simulink model "dextair_mechanics_without_spring"  (R2018b)
settings: Solver=VariableStepAuto  StartTime=0.0  StopTime=100  RelTol=1e-3  EnableMultiTasking=on
values from neighbouring files (symbols this model uses):
  a = 1.7*10^(-6)    (= 1.7e-06)    [MAIN.m]
  delta = 0.32    [MAIN.m]
  g = 9.8    [MAIN.m]
  k = 0    [MAIN.m]
  L = 0.16    [MAIN.m]
  l_0 = 10    [MAIN.m]
  m = 2.07    [MAIN.m]
  PID_D_phi = PID_D    (= 19)    [MAIN.m]
  PID_D_psi = PID_D    (= 19)    [MAIN.m]
  PID_D_theta = PID_D    (= 19)    [MAIN.m]
  PID_D_x = PID_D    (= 19)    [MAIN.m]
  PID_D_y = PID_D    (= 19)    [MAIN.m]
  PID_D_z = PID_D    (= 19)    [MAIN.m]
  PID_I_phi = PID_I    (= 2.12)    [MAIN.m]
  PID_I_psi = PID_I    (= 2.12)    [MAIN.m]
  PID_I_theta = PID_I    (= 2.12)    [MAIN.m]
  PID_I_x = PID_I    (= 2.12)    [MAIN.m]
  PID_I_y = PID_I    (= 2.12)    [MAIN.m]
  PID_I_z = PID_I    (= 2.12)    [MAIN.m]
  PID_P_phi = PID_P    (= 12.71)    [MAIN.m]
  PID_P_psi = PID_P    (= 12.71)    [MAIN.m]
  PID_P_theta = PID_P    (= 12.71)    [MAIN.m]
  PID_P_x = PID_P    (= 12.71)    [MAIN.m]
  PID_P_y = PID_P    (= 12.71)    [MAIN.m]
  PID_P_z = PID_P    (= 12.71)    [MAIN.m]
  s = tf('s')    [MAIN.m]
  xl = 0.01    [MAIN.m]
  Z_0 = m*g/k+l_0    [MAIN.m]
undefined symbols (not defined in the file or in its folder): X, Y, Z
libraries: sm_lib x28, nesl_utility x11, simulink x7
(part 1 of 2)
settings Model: Creator=shaabang  LastModifiedBy=shaabang
settings DataIOCC: LimitDataPoints=on
settings OptimizationCC: LifeSpan=inf
settings DebuggingCC: AllowSymbolicDim=off  SFUnexpectedBacktrackingDiag=warning  SFNoUnconditionalDefaultTransitionDiag=warning  SFExecutionAtInitializationDiag=none
settings SFSimCC: SimUseLocalCustomCode=off
settings RTWCC: RTWUseLocalCustomCode=off
settings CodeAppCC: StateflowObjectComments=on
settings GRTTargetCC: TargetLangStandard=C89/C90 (ANSI)  GeneratePreprocessorConditionals=Disable all
settings ConfigComp: CovMetricSettings=dw  CovHtmlReporting=on  CovSaveCumulativeToWorkspaceVar=on  CovSaveSingleToWorkspaceVar=on  CovExternalEMLEnable=off  CovSFcnEnable=off
settings SimscapeCC: SimscapeNominalValues="[{\"value\":\"10\",\"unit\":\"V\"},{\"value\":\"1\",\"unit\":\"A\"},{\"value\":\"10\",\"unit\":\"N*m\"},{\"value\":\"10\",\"unit\":\"bar\"},{\"value\":\"100\",\"unit\":\"kJ/kg\"},{\"value\":\"1\",\"unit\":\"kW\"},{\"value\":\"300\",\"unit\":\"K\"},{\"value\":\"100\",\"unit\":\"cm^3/s\"},{\"value\":\"1\",\"unit\":\"kN\"},{\"value\":\"1\",\"unit\":\"g/cm^3\"},{\"value\":\"1\",\"unit\":\"l\"},{\"value\":\"1\",\"unit\":\"cm^2\"},{\"value\":\"60\",\"unit\":\"Hz\"}]"  SimscapeLogType=all  SimscapeLogDataHistory=10000
settings ConfigurationSet: Description=SimMechanics 2G

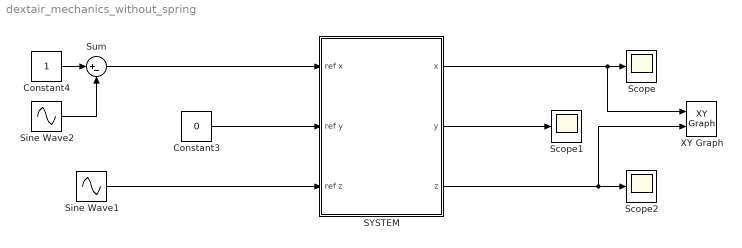
== system dextair_mechanics_without_spring ==
  Constant3 : Constant  Value=0
  Constant4 : Constant
  SYSTEM : Subsystem
  Scope : Scope
  Scope1 : Scope
  Scope2 : Scope
  Sine Wave1 : Sin  Frequency=0.5  SampleTime=0
  Sine Wave2 : Sin  Frequency=0.5  Phase=pi/2  SampleTime=0
  Sum : Sum  Inputs=|+-
  XY Graph : simulink/Sinks/XY Graph  xmin=-0.5  xmax=2.5  ymin=-1.5  ymax=1.5  st=-1
  wires:
  Sum/1 -> SYSTEM/1(ref x)
  SYSTEM/1(x) -> XY Graph/1, Scope/1
  Sine Wave1/1 -> SYSTEM/3(ref z)
  SYSTEM/2(y) -> Scope1/1
  Constant4/1 -> Sum/1
  Constant3/1 -> SYSTEM/2(ref y)
  SYSTEM/3(z) -> XY Graph/2, Scope2/1
  Sine Wave2/1 -> Sum/2

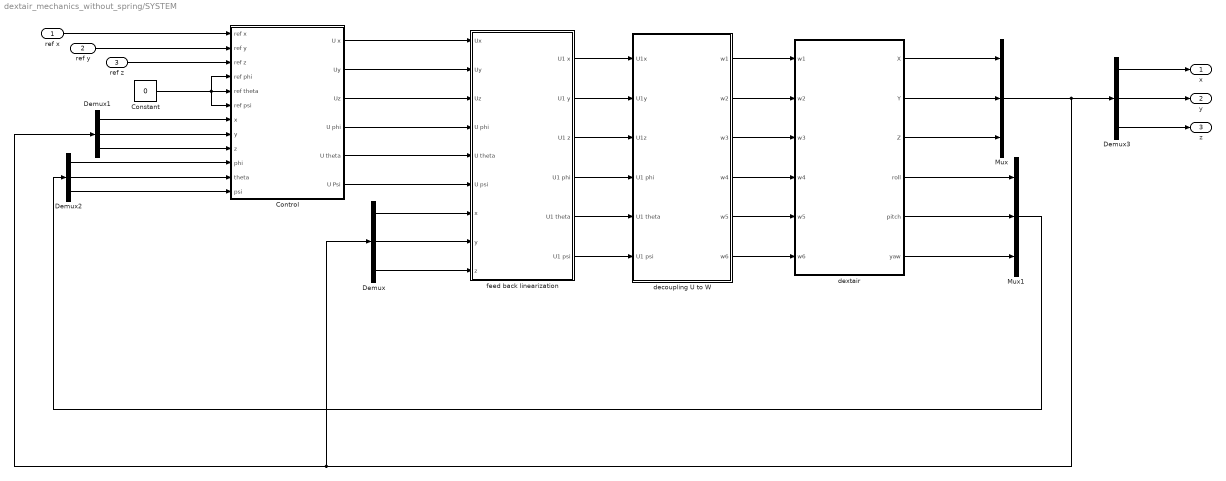
== system dextair_mechanics_without_spring/SYSTEM ==
  ref x : Inport
  ref y : Inport  Port=2
  ref z : Inport  Port=3
  Constant : Constant  Value=0
  Control : Subsystem
  Demux{,1..3} (4 alike) : Demux  Outputs=3
  Mux : Mux  Inputs=3
  Mux1 : Mux  Inputs=3
  decoupling U to W : Subsystem
  dextair : Subsystem
  feed back linearization : Subsystem
  x : Outport
  y : Outport  Port=2
  z : Outport  Port=3
  wires:
  decoupling U to W/5(w5) -> dextair/5(w5)
  Demux1/2 -> Control/8(y)
  feed back linearization/2(U1 y) -> decoupling U to W/2(U1y)
  ref y/1 -> Control/2(ref y)
  Control/2(Uy) -> feed back linearization/2(Uy)
  feed back linearization/5(U1 theta) -> decoupling U to W/5(U1 theta)
  decoupling U to W/2(w2) -> dextair/2(w2)
  decoupling U to W/4(w4) -> dextair/4(w4)
  dextair/5(pitch) -> Mux1/2
  Control/6(U Psi) -> feed back linearization/6(U psi)
  dextair/1(X) -> Mux/1
  Control/5(U theta) -> feed back linearization/5(U theta)
  Demux2/2 -> Control/11(theta)
  decoupling U to W/6(w6) -> dextair/6(w6)
  feed back linearization/3(U1 z) -> decoupling U to W/3(U1z)
  Demux1/1 -> Control/7(x)
  Demux2/3 -> Control/12(psi)
  decoupling U to W/1(w1) -> dextair/1(w1)
  Demux/1 -> feed back linearization/7(x)
  Control/4(U phi) -> feed back linearization/4(U phi)
  Control/3(Uz) -> feed back linearization/3(Uz)
  Constant/1 -> Control/6(ref psi), Control/4(ref phi), Control/5(ref theta)
  Demux2/1 -> Control/10(phi)
  dextair/4(roll) -> Mux1/1
  Demux1/3 -> Control/9(z)
  dextair/6(yaw) -> Mux1/3
  Control/1(U x) -> feed back linearization/1(Ux)
  feed back linearization/6(U1 psi) -> decoupling U to W/6(U1 psi)
  ref x/1 -> Control/1(ref x)
  dextair/3(Z) -> Mux/3
  ref z/1 -> Control/3(ref z)
  Demux3/2 -> y/1
  Demux/2 -> feed back linearization/8(y)
  Demux3/3 -> z/1
  Demux3/1 -> x/1
  dextair/2(Y) -> Mux/2
  feed back linearization/1(U1 x) -> decoupling U to W/1(U1x)
  feed back linearization/4(U1 phi) -> decoupling U to W/4(U1 phi)
  Demux/3 -> feed back linearization/9(z)
  decoupling U to W/3(w3) -> dextair/3(w3)
  Mux1/1 -> Demux2/1
  Mux/1 -> Demux/1, Demux1/1, Demux3/1

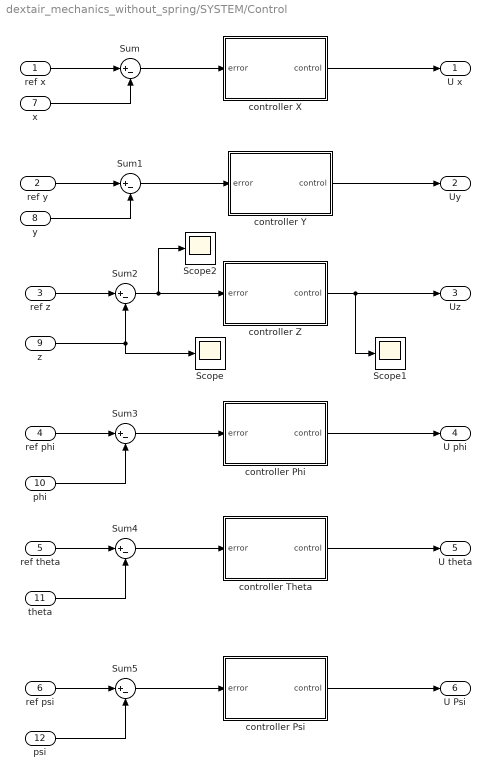
== system dextair_mechanics_without_spring/SYSTEM/Control ==
  ref x : Inport
  ref y : Inport  Port=2
  ref z : Inport  Port=3
  ref phi : Inport  Port=4
  ref theta : Inport  Port=5
  ref psi : Inport  Port=6
  x : Inport  Port=7
  y : Inport  Port=8
  z : Inport  Port=9
  phi : Inport  Port=10
  theta : Inport  Port=11
  psi : Inport  Port=12
  Scope : Scope
  Scope1 : Scope
  Scope2 : Scope
  Sum{,1..5} (6 alike) : Sum  Inputs=|+-
  controller Phi : Subsystem
  controller Psi : Subsystem
  controller Theta : Subsystem
  controller X : Subsystem
  controller Y : Subsystem
  controller Z : Subsystem
  U x : Outport
  Uy : Outport  Port=2
  Uz : Outport  Port=3
  U phi : Outport  Port=4
  U theta : Outport  Port=5
  U Psi : Outport  Port=6
  wires:
  ref psi/1 -> Sum5/1
  theta/1 -> Sum4/2
  z/1 -> Scope/1, Sum2/2
  ref phi/1 -> Sum3/1
  x/1 -> Sum/2
  Sum/1 -> controller X/1("error ")
  Sum3/1 -> controller Phi/1("error ")
  controller X/1("control ") -> U x/1
  Sum4/1 -> controller Theta/1("error ")
  Sum2/1 -> Scope2/1, controller Z/1("error ")
  y/1 -> Sum1/2
  Sum1/1 -> controller Y/1("error ")
  controller Phi/1("control ") -> U phi/1
  ref theta/1 -> Sum4/1
  controller Y/1("control ") -> Uy/1
  controller Psi/1("control ") -> U Psi/1
  psi/1 -> Sum5/2
  controller Z/1("control ") -> Scope1/1, Uz/1
  ref z/1 -> Sum2/1
  phi/1 -> Sum3/2
  controller Theta/1("control ") -> U theta/1
  Sum5/1 -> controller Psi/1("error ")
  ref x/1 -> Sum/1
  ref y/1 -> Sum1/1

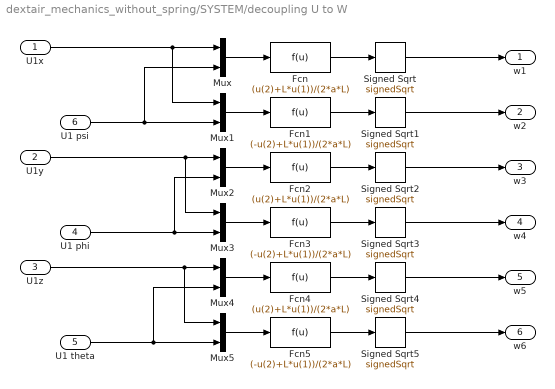
== system dextair_mechanics_without_spring/SYSTEM/decoupling U to W ==
  U1x : Inport
  U1y : Inport  Port=2
  U1z : Inport  Port=3
  U1 phi : Inport  Port=4
  U1 theta : Inport  Port=5
  U1 psi : Inport  Port=6
  Fcn : Fcn  Expr=(u(2)+L*u(1))/(2*a*L)
  Fcn1 : Fcn  Expr=(-u(2)+L*u(1))/(2*a*L)
  Fcn2 : Fcn  Expr=(u(2)+L*u(1))/(2*a*L)
  Fcn3 : Fcn  Expr=(-u(2)+L*u(1))/(2*a*L)
  Fcn4 : Fcn  Expr=(u(2)+L*u(1))/(2*a*L)
  Fcn5 : Fcn  Expr=(-u(2)+L*u(1))/(2*a*L)
  Mux{,1..5} (6 alike) : Mux  Inputs=2
  Signed Sqrt{,1..5} (6 alike) : Sqrt  Operator=signedSqrt  SaturateOnIntegerOverflow=on
  w1 : Outport
  w2 : Outport  Port=2
  w3 : Outport  Port=3
  w4 : Outport  Port=4
  w5 : Outport  Port=5
  w6 : Outport  Port=6
  wires:
  Mux2/1 -> Fcn2/1
  Mux1/1 -> Fcn1/1
  Fcn5/1 -> Signed Sqrt5/1
  U1z/1 -> Mux5/1, Mux4/1
  Fcn3/1 -> Signed Sqrt3/1
  U1 theta/1 -> Mux4/2, Mux5/2
  Signed Sqrt2/1 -> w3/1
  Fcn/1 -> Signed Sqrt/1
  Mux3/1 -> Fcn3/1
  U1 psi/1 -> Mux/2, Mux1/2
  Fcn2/1 -> Signed Sqrt2/1
  Signed Sqrt4/1 -> w5/1
  Signed Sqrt5/1 -> w6/1
  Fcn1/1 -> Signed Sqrt1/1
  Signed Sqrt3/1 -> w4/1
  Signed Sqrt1/1 -> w2/1
  Mux/1 -> Fcn/1
  U1 phi/1 -> Mux2/2, Mux3/2
  U1x/1 -> Mux1/1, Mux/1
  U1y/1 -> Mux3/1, Mux2/1
  Mux5/1 -> Fcn5/1
  Fcn4/1 -> Signed Sqrt4/1
  Signed Sqrt/1 -> w1/1
  Mux4/1 -> Fcn4/1

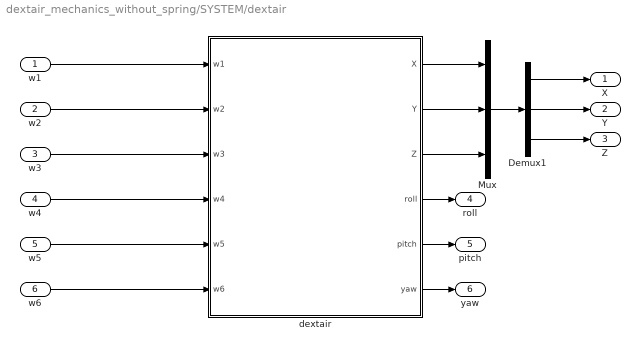
== system dextair_mechanics_without_spring/SYSTEM/dextair ==
  w1 : Inport
  w2 : Inport  Port=2
  w3 : Inport  Port=3
  w4 : Inport  Port=4
  w5 : Inport  Port=5
  w6 : Inport  Port=6
  Demux1 : Demux  Outputs=3
  Mux : Mux  Inputs=3
  dextair : Subsystem
  X : Outport
  Y : Outport  Port=2
  Z : Outport  Port=3
  roll : Outport  Port=4
  pitch : Outport  Port=5
  yaw : Outport  Port=6
  wires:
  Demux1/3 -> Z/1
  Demux1/1 -> X/1
  dextair/6(yaw) -> yaw/1
  w3/1 -> dextair/3(w3)
  dextair/4(roll) -> roll/1
  Demux1/2 -> Y/1
  dextair/2(Y) -> Mux/2
  dextair/3(Z) -> Mux/3
  dextair/5(pitch) -> pitch/1
  dextair/1(X) -> Mux/1
  w2/1 -> dextair/2(w2)
  w4/1 -> dextair/4(w4)
  Mux/1 -> Demux1/1
  w6/1 -> dextair/6(w6)
  w5/1 -> dextair/5(w5)
  w1/1 -> dextair/1(w1)

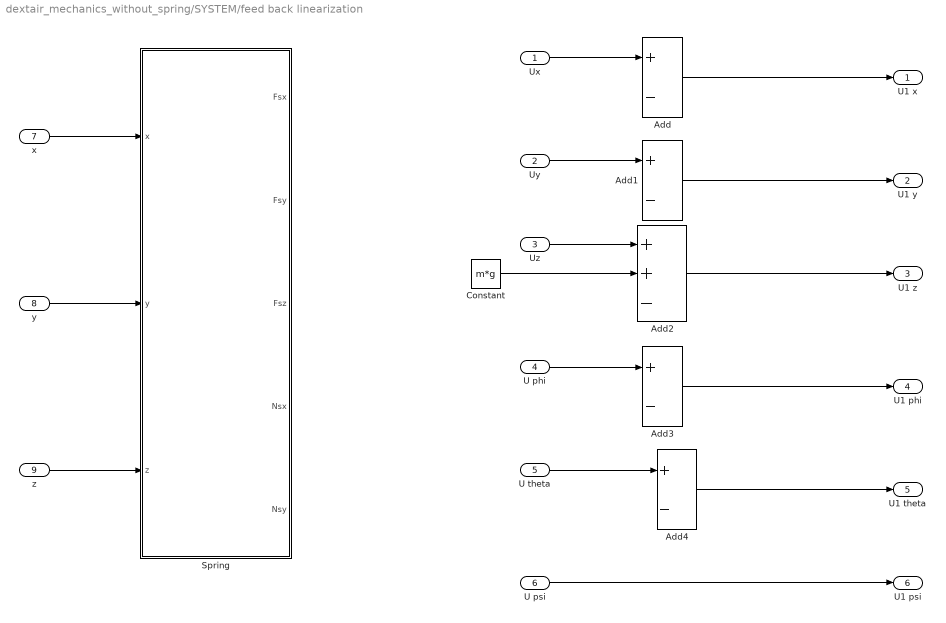
== system dextair_mechanics_without_spring/SYSTEM/feed back linearization ==
  Ux : Inport
  Uy : Inport  Port=2
  Uz : Inport  Port=3
  U phi : Inport  Port=4
  U theta : Inport  Port=5
  U psi : Inport  Port=6
  x : Inport  Port=7
  y : Inport  Port=8
  z : Inport  Port=9
  Add{,1,3..4} (4 alike) : Sum  Inputs=+-
  Add2 : Sum  Inputs=++-
  Constant : Constant  Value=m*g
  Spring : Subsystem
  U1 x : Outport
  U1 y : Outport  Port=2
  U1 z : Outport  Port=3
  U1 phi : Outport  Port=4
  U1 theta : Outport  Port=5
  U1 psi : Outport  Port=6
  wires:
  U psi/1 -> U1 psi/1
  Add/1 -> U1 x/1
  Uy/1 -> Add1/1
  z/1 -> Spring/3(z)
  y/1 -> Spring/2(y)
  Constant/1 -> Add2/2
  U phi/1 -> Add3/1
  Add2/1 -> U1 z/1
  Add4/1 -> U1 theta/1
  U theta/1 -> Add4/1
  x/1 -> Spring/1(x)
  Ux/1 -> Add/1
  Add1/1 -> U1 y/1
  Add3/1 -> U1 phi/1
  Uz/1 -> Add2/1

== system dextair_mechanics_without_spring/SYSTEM/Control/controller Phi ==
  "error " : Inport
  PID Controller : simulink/Continuous/PID Controller  Controller=PID  Form=Parallel  TimeDomain=Continuous-time  SampleTime=-1  IntegratorMethod=Forward Euler  FilterMethod=Forward Euler  ControllerParametersSource=internal  P=PID_P_phi  I=PID_I_phi  D=PID_D_phi  UseFilter=on  N=100  TunerSelectOption=Transfer Function Based (PID Tuner App)  InitialConditionSource=internal  InitialConditionForIntegrator=0  InitialConditionForFilter=0  DifferentiatorICPrevScaledInput=0  ExternalReset=none  TrackingMode=off  Kt=1  LimitOutput=off  UpperSaturationLimit=inf  LowerSaturationLimit=-inf  LinearizeAsGain=on  AntiWindupMode=none  Kb=1  POutMin=[]  POutMax=[]  IOutMin=[]  IOutMax=[]  DOutMin=[]  DOutMax=[]  NOutMin=[]  NOutMax=[]  SumOutMin=[]  SumOutMax=[]  SaturationOutMin=[]  SaturationOutMax=[]  PParamMin=[]  PParamMax=[]  IParamMin=[]  IParamMax=[]  DParamMin=[]  DParamMax=[]  NParamMin=[]  NParamMax=[]  KbParamMin=[]  KbParamMax=[]  KtParamMin=[]  KtParamMax=[]  KbOutMin=[]  KbOutMax=[]  KtOutMin=[]  KtOutMax=[]  IntegratorOutMin=[]  IntegratorOutMax=[]  FilterOutMin=[]  FilterOutMax=[]  SumI1OutMin=[]  SumI1OutMax=[]  SumI2OutMin=[]  SumI2OutMax=[]  SumI3OutMin=[]  SumI3OutMax=[]  SumI4OutMin=[]  SumI4OutMax=[]  SumDOutMin=[]  SumDOutMax=[]  DifferentiatorOutMin=[]  DifferentiatorOutMax=[]  FilterDiffOutCoefMin=[]  FilterDiffOutCoefMax=[]  ReciprocalOutMin=[]  ReciprocalOutMax=[]  SumDenOutMin=[]  SumDenOutMax=[]  SumNumOutMin=[]  SumNumOutMax=[]  DivideOutMin=[]  DivideOutMax=[]  IntegratorContinuousStateAttributes=''  IntegratorStateMustResolveToSignalObject=off  IntegratorRTWStateStorageClass=Auto  FilterContinuousStateAttributes=''  FilterStateMustResolveToSignalObject=off  FilterRTWStateStorageClass=Auto  ParallelPVariant=InternalParameters  IdealPVariant=Disabled  IVariant=InternalParameters  DVariant=InternalParameters  IntegratorVariant=Continuous  SatVariant=Disabled  AWVariant=Passthrough  PCopyVariant=Disabled  TRVariant=Disabled  FdbkBlocksVariant=Forward  IdealPFdbkVariant=Disabled  SatFdbkVariant=Disabled  DerivativeFilterVariant=ContFilter  NVariant=InternalParameters  NCopyVariant=Disabled  FilterICVariant=InternalICsFilter  IntegratorICVariant=InternalICs  ExternalResetVariant=Disabled  TRSumVariant=Passthrough  SumFdbkVariant=Disabled  SumVariant=Sum_PID
  "control " : Outport
  wires:
  PID Controller/1 -> "control "/1
  "error "/1 -> PID Controller/1

== system dextair_mechanics_without_spring/SYSTEM/Control/controller Psi ==
  "error " : Inport
  PID Controller : simulink/Continuous/PID Controller  Controller=PID  Form=Parallel  TimeDomain=Continuous-time  SampleTime=-1  IntegratorMethod=Forward Euler  FilterMethod=Forward Euler  ControllerParametersSource=internal  P=PID_P_psi  I=PID_I_psi  D=PID_D_psi  UseFilter=on  N=100  TunerSelectOption=Transfer Function Based (PID Tuner App)  InitialConditionSource=internal  InitialConditionForIntegrator=0  InitialConditionForFilter=0  DifferentiatorICPrevScaledInput=0  ExternalReset=none  TrackingMode=off  Kt=1  LimitOutput=off  UpperSaturationLimit=inf  LowerSaturationLimit=-inf  LinearizeAsGain=on  AntiWindupMode=none  Kb=1  POutMin=[]  POutMax=[]  IOutMin=[]  IOutMax=[]  DOutMin=[]  DOutMax=[]  NOutMin=[]  NOutMax=[]  SumOutMin=[]  SumOutMax=[]  SaturationOutMin=[]  SaturationOutMax=[]  PParamMin=[]  PParamMax=[]  IParamMin=[]  IParamMax=[]  DParamMin=[]  DParamMax=[]  NParamMin=[]  NParamMax=[]  KbParamMin=[]  KbParamMax=[]  KtParamMin=[]  KtParamMax=[]  KbOutMin=[]  KbOutMax=[]  KtOutMin=[]  KtOutMax=[]  IntegratorOutMin=[]  IntegratorOutMax=[]  FilterOutMin=[]  FilterOutMax=[]  SumI1OutMin=[]  SumI1OutMax=[]  SumI2OutMin=[]  SumI2OutMax=[]  SumI3OutMin=[]  SumI3OutMax=[]  SumI4OutMin=[]  SumI4OutMax=[]  SumDOutMin=[]  SumDOutMax=[]  DifferentiatorOutMin=[]  DifferentiatorOutMax=[]  FilterDiffOutCoefMin=[]  FilterDiffOutCoefMax=[]  ReciprocalOutMin=[]  ReciprocalOutMax=[]  SumDenOutMin=[]  SumDenOutMax=[]  SumNumOutMin=[]  SumNumOutMax=[]  DivideOutMin=[]  DivideOutMax=[]  IntegratorContinuousStateAttributes=''  IntegratorStateMustResolveToSignalObject=off  IntegratorRTWStateStorageClass=Auto  FilterContinuousStateAttributes=''  FilterStateMustResolveToSignalObject=off  FilterRTWStateStorageClass=Auto  ParallelPVariant=InternalParameters  IdealPVariant=Disabled  IVariant=InternalParameters  DVariant=InternalParameters  IntegratorVariant=Continuous  SatVariant=Disabled  AWVariant=Passthrough  PCopyVariant=Disabled  TRVariant=Disabled  FdbkBlocksVariant=Forward  IdealPFdbkVariant=Disabled  SatFdbkVariant=Disabled  DerivativeFilterVariant=ContFilter  NVariant=InternalParameters  NCopyVariant=Disabled  FilterICVariant=InternalICsFilter  IntegratorICVariant=InternalICs  ExternalResetVariant=Disabled  TRSumVariant=Passthrough  SumFdbkVariant=Disabled  SumVariant=Sum_PID
  "control " : Outport
  wires:
  PID Controller/1 -> "control "/1
  "error "/1 -> PID Controller/1

== system dextair_mechanics_without_spring/SYSTEM/Control/controller Theta ==
  "error " : Inport
  PID Controller : simulink/Continuous/PID Controller  Controller=PID  Form=Parallel  TimeDomain=Continuous-time  SampleTime=-1  IntegratorMethod=Forward Euler  FilterMethod=Forward Euler  ControllerParametersSource=internal  P=PID_P_theta  I=PID_I_theta  D=PID_D_theta  UseFilter=on  N=100  TunerSelectOption=Transfer Function Based (PID Tuner App)  InitialConditionSource=internal  InitialConditionForIntegrator=0  InitialConditionForFilter=0  DifferentiatorICPrevScaledInput=0  ExternalReset=none  TrackingMode=off  Kt=1  LimitOutput=off  UpperSaturationLimit=inf  LowerSaturationLimit=-inf  LinearizeAsGain=on  AntiWindupMode=none  Kb=1  POutMin=[]  POutMax=[]  IOutMin=[]  IOutMax=[]  DOutMin=[]  DOutMax=[]  NOutMin=[]  NOutMax=[]  SumOutMin=[]  SumOutMax=[]  SaturationOutMin=[]  SaturationOutMax=[]  PParamMin=[]  PParamMax=[]  IParamMin=[]  IParamMax=[]  DParamMin=[]  DParamMax=[]  NParamMin=[]  NParamMax=[]  KbParamMin=[]  KbParamMax=[]  KtParamMin=[]  KtParamMax=[]  KbOutMin=[]  KbOutMax=[]  KtOutMin=[]  KtOutMax=[]  IntegratorOutMin=[]  IntegratorOutMax=[]  FilterOutMin=[]  FilterOutMax=[]  SumI1OutMin=[]  SumI1OutMax=[]  SumI2OutMin=[]  SumI2OutMax=[]  SumI3OutMin=[]  SumI3OutMax=[]  SumI4OutMin=[]  SumI4OutMax=[]  SumDOutMin=[]  SumDOutMax=[]  DifferentiatorOutMin=[]  DifferentiatorOutMax=[]  FilterDiffOutCoefMin=[]  FilterDiffOutCoefMax=[]  ReciprocalOutMin=[]  ReciprocalOutMax=[]  SumDenOutMin=[]  SumDenOutMax=[]  SumNumOutMin=[]  SumNumOutMax=[]  DivideOutMin=[]  DivideOutMax=[]  IntegratorContinuousStateAttributes=''  IntegratorStateMustResolveToSignalObject=off  IntegratorRTWStateStorageClass=Auto  FilterContinuousStateAttributes=''  FilterStateMustResolveToSignalObject=off  FilterRTWStateStorageClass=Auto  ParallelPVariant=InternalParameters  IdealPVariant=Disabled  IVariant=InternalParameters  DVariant=InternalParameters  IntegratorVariant=Continuous  SatVariant=Disabled  AWVariant=Passthrough  PCopyVariant=Disabled  TRVariant=Disabled  FdbkBlocksVariant=Forward  IdealPFdbkVariant=Disabled  SatFdbkVariant=Disabled  DerivativeFilterVariant=ContFilter  NVariant=InternalParameters  NCopyVariant=Disabled  FilterICVariant=InternalICsFilter  IntegratorICVariant=InternalICs  ExternalResetVariant=Disabled  TRSumVariant=Passthrough  SumFdbkVariant=Disabled  SumVariant=Sum_PID
  "control " : Outport
  wires:
  PID Controller/1 -> "control "/1
  "error "/1 -> PID Controller/1

== system dextair_mechanics_without_spring/SYSTEM/Control/controller X ==
  "error " : Inport
  PID Controller : simulink/Continuous/PID Controller  Controller=PID  Form=Parallel  TimeDomain=Continuous-time  SampleTime=-1  IntegratorMethod=Forward Euler  FilterMethod=Forward Euler  ControllerParametersSource=internal  P=PID_P_x  I=PID_I_x  D=PID_D_x  UseFilter=on  N=100  TunerSelectOption=Transfer Function Based (PID Tuner App)  InitialConditionSource=internal  InitialConditionForIntegrator=0  InitialConditionForFilter=0  DifferentiatorICPrevScaledInput=0  ExternalReset=none  TrackingMode=off  Kt=1  LimitOutput=off  UpperSaturationLimit=inf  LowerSaturationLimit=-inf  LinearizeAsGain=on  AntiWindupMode=none  Kb=1  POutMin=[]  POutMax=[]  IOutMin=[]  IOutMax=[]  DOutMin=[]  DOutMax=[]  NOutMin=[]  NOutMax=[]  SumOutMin=[]  SumOutMax=[]  SaturationOutMin=[]  SaturationOutMax=[]  PParamMin=[]  PParamMax=[]  IParamMin=[]  IParamMax=[]  DParamMin=[]  DParamMax=[]  NParamMin=[]  NParamMax=[]  KbParamMin=[]  KbParamMax=[]  KtParamMin=[]  KtParamMax=[]  KbOutMin=[]  KbOutMax=[]  KtOutMin=[]  KtOutMax=[]  IntegratorOutMin=[]  IntegratorOutMax=[]  FilterOutMin=[]  FilterOutMax=[]  SumI1OutMin=[]  SumI1OutMax=[]  SumI2OutMin=[]  SumI2OutMax=[]  SumI3OutMin=[]  SumI3OutMax=[]  SumI4OutMin=[]  SumI4OutMax=[]  SumDOutMin=[]  SumDOutMax=[]  DifferentiatorOutMin=[]  DifferentiatorOutMax=[]  FilterDiffOutCoefMin=[]  FilterDiffOutCoefMax=[]  ReciprocalOutMin=[]  ReciprocalOutMax=[]  SumDenOutMin=[]  SumDenOutMax=[]  SumNumOutMin=[]  SumNumOutMax=[]  DivideOutMin=[]  DivideOutMax=[]  IntegratorContinuousStateAttributes=''  IntegratorStateMustResolveToSignalObject=off  IntegratorRTWStateStorageClass=Auto  FilterContinuousStateAttributes=''  FilterStateMustResolveToSignalObject=off  FilterRTWStateStorageClass=Auto  ParallelPVariant=InternalParameters  IdealPVariant=Disabled  IVariant=InternalParameters  DVariant=InternalParameters  IntegratorVariant=Continuous  SatVariant=Disabled  AWVariant=Passthrough  PCopyVariant=Disabled  TRVariant=Disabled  FdbkBlocksVariant=Forward  IdealPFdbkVariant=Disabled  SatFdbkVariant=Disabled  DerivativeFilterVariant=ContFilter  NVariant=InternalParameters  NCopyVariant=Disabled  FilterICVariant=InternalICsFilter  IntegratorICVariant=InternalICs  ExternalResetVariant=Disabled  TRSumVariant=Passthrough  SumFdbkVariant=Disabled  SumVariant=Sum_PID
  "control " : Outport
  wires:
  PID Controller/1 -> "control "/1
  "error "/1 -> PID Controller/1

== system dextair_mechanics_without_spring/SYSTEM/Control/controller Y ==
  "error " : Inport
  PID Controller : simulink/Continuous/PID Controller  Controller=PID  Form=Parallel  TimeDomain=Continuous-time  SampleTime=-1  IntegratorMethod=Forward Euler  FilterMethod=Forward Euler  ControllerParametersSource=internal  P=PID_P_y  I=PID_I_y  D=PID_D_y  UseFilter=on  N=100  TunerSelectOption=Transfer Function Based (PID Tuner App)  InitialConditionSource=internal  InitialConditionForIntegrator=0  InitialConditionForFilter=0  DifferentiatorICPrevScaledInput=0  ExternalReset=none  TrackingMode=off  Kt=1  LimitOutput=off  UpperSaturationLimit=inf  LowerSaturationLimit=-inf  LinearizeAsGain=on  AntiWindupMode=none  Kb=1  POutMin=[]  POutMax=[]  IOutMin=[]  IOutMax=[]  DOutMin=[]  DOutMax=[]  NOutMin=[]  NOutMax=[]  SumOutMin=[]  SumOutMax=[]  SaturationOutMin=[]  SaturationOutMax=[]  PParamMin=[]  PParamMax=[]  IParamMin=[]  IParamMax=[]  DParamMin=[]  DParamMax=[]  NParamMin=[]  NParamMax=[]  KbParamMin=[]  KbParamMax=[]  KtParamMin=[]  KtParamMax=[]  KbOutMin=[]  KbOutMax=[]  KtOutMin=[]  KtOutMax=[]  IntegratorOutMin=[]  IntegratorOutMax=[]  FilterOutMin=[]  FilterOutMax=[]  SumI1OutMin=[]  SumI1OutMax=[]  SumI2OutMin=[]  SumI2OutMax=[]  SumI3OutMin=[]  SumI3OutMax=[]  SumI4OutMin=[]  SumI4OutMax=[]  SumDOutMin=[]  SumDOutMax=[]  DifferentiatorOutMin=[]  DifferentiatorOutMax=[]  FilterDiffOutCoefMin=[]  FilterDiffOutCoefMax=[]  ReciprocalOutMin=[]  ReciprocalOutMax=[]  SumDenOutMin=[]  SumDenOutMax=[]  SumNumOutMin=[]  SumNumOutMax=[]  DivideOutMin=[]  DivideOutMax=[]  IntegratorContinuousStateAttributes=''  IntegratorStateMustResolveToSignalObject=off  IntegratorRTWStateStorageClass=Auto  FilterContinuousStateAttributes=''  FilterStateMustResolveToSignalObject=off  FilterRTWStateStorageClass=Auto  ParallelPVariant=InternalParameters  IdealPVariant=Disabled  IVariant=InternalParameters  DVariant=InternalParameters  IntegratorVariant=Continuous  SatVariant=Disabled  AWVariant=Passthrough  PCopyVariant=Disabled  TRVariant=Disabled  FdbkBlocksVariant=Forward  IdealPFdbkVariant=Disabled  SatFdbkVariant=Disabled  DerivativeFilterVariant=ContFilter  NVariant=InternalParameters  NCopyVariant=Disabled  FilterICVariant=InternalICsFilter  IntegratorICVariant=InternalICs  ExternalResetVariant=Disabled  TRSumVariant=Passthrough  SumFdbkVariant=Disabled  SumVariant=Sum_PID
  "control " : Outport
  wires:
  "error "/1 -> PID Controller/1
  PID Controller/1 -> "control "/1

== system dextair_mechanics_without_spring/SYSTEM/Control/controller Z ==
  "error " : Inport
  PID Controller : simulink/Continuous/PID Controller  Controller=PID  Form=Parallel  TimeDomain=Continuous-time  SampleTime=-1  IntegratorMethod=Forward Euler  FilterMethod=Forward Euler  ControllerParametersSource=internal  P=PID_P_z  I=PID_I_z  D=PID_D_z  UseFilter=on  N=100  TunerSelectOption=Transfer Function Based (PID Tuner App)  InitialConditionSource=internal  InitialConditionForIntegrator=0  InitialConditionForFilter=0  DifferentiatorICPrevScaledInput=0  ExternalReset=none  TrackingMode=off  Kt=1  LimitOutput=off  UpperSaturationLimit=inf  LowerSaturationLimit=-inf  LinearizeAsGain=on  AntiWindupMode=none  Kb=1  POutMin=[]  POutMax=[]  IOutMin=[]  IOutMax=[]  DOutMin=[]  DOutMax=[]  NOutMin=[]  NOutMax=[]  SumOutMin=[]  SumOutMax=[]  SaturationOutMin=[]  SaturationOutMax=[]  PParamMin=[]  PParamMax=[]  IParamMin=[]  IParamMax=[]  DParamMin=[]  DParamMax=[]  NParamMin=[]  NParamMax=[]  KbParamMin=[]  KbParamMax=[]  KtParamMin=[]  KtParamMax=[]  KbOutMin=[]  KbOutMax=[]  KtOutMin=[]  KtOutMax=[]  IntegratorOutMin=[]  IntegratorOutMax=[]  FilterOutMin=[]  FilterOutMax=[]  SumI1OutMin=[]  SumI1OutMax=[]  SumI2OutMin=[]  SumI2OutMax=[]  SumI3OutMin=[]  SumI3OutMax=[]  SumI4OutMin=[]  SumI4OutMax=[]  SumDOutMin=[]  SumDOutMax=[]  DifferentiatorOutMin=[]  DifferentiatorOutMax=[]  FilterDiffOutCoefMin=[]  FilterDiffOutCoefMax=[]  ReciprocalOutMin=[]  ReciprocalOutMax=[]  SumDenOutMin=[]  SumDenOutMax=[]  SumNumOutMin=[]  SumNumOutMax=[]  DivideOutMin=[]  DivideOutMax=[]  IntegratorContinuousStateAttributes=''  IntegratorStateMustResolveToSignalObject=off  IntegratorRTWStateStorageClass=Auto  FilterContinuousStateAttributes=''  FilterStateMustResolveToSignalObject=off  FilterRTWStateStorageClass=Auto  ParallelPVariant=InternalParameters  IdealPVariant=Disabled  IVariant=InternalParameters  DVariant=InternalParameters  IntegratorVariant=Continuous  SatVariant=Disabled  AWVariant=Passthrough  PCopyVariant=Disabled  TRVariant=Disabled  FdbkBlocksVariant=Forward  IdealPFdbkVariant=Disabled  SatFdbkVariant=Disabled  DerivativeFilterVariant=ContFilter  NVariant=InternalParameters  NCopyVariant=Disabled  FilterICVariant=InternalICsFilter  IntegratorICVariant=InternalICs  ExternalResetVariant=Disabled  TRSumVariant=Passthrough  SumFdbkVariant=Disabled  SumVariant=Sum_PID
  "control " : Outport
  wires:
  PID Controller/1 -> "control "/1
  "error "/1 -> PID Controller/1
